simulink model ""  (R2025b)
settings: Solver=FixedStepAuto  StartTime=0.0  StopTime=inf  FixedStep=0.01  RelTol=1e-3
undefined symbols (not defined in the file or in its folder): LF
libraries: instrumentseriallib x4, simulink x1
settings Model: Creator=talles  LastModifiedBy=a_jax

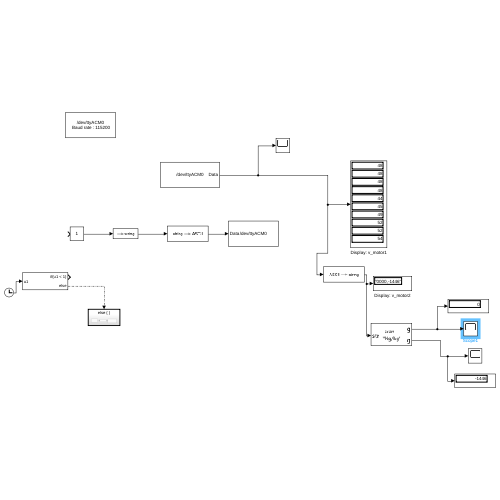
[thumbnail: Simulink's stored preview of the top-level diagram]
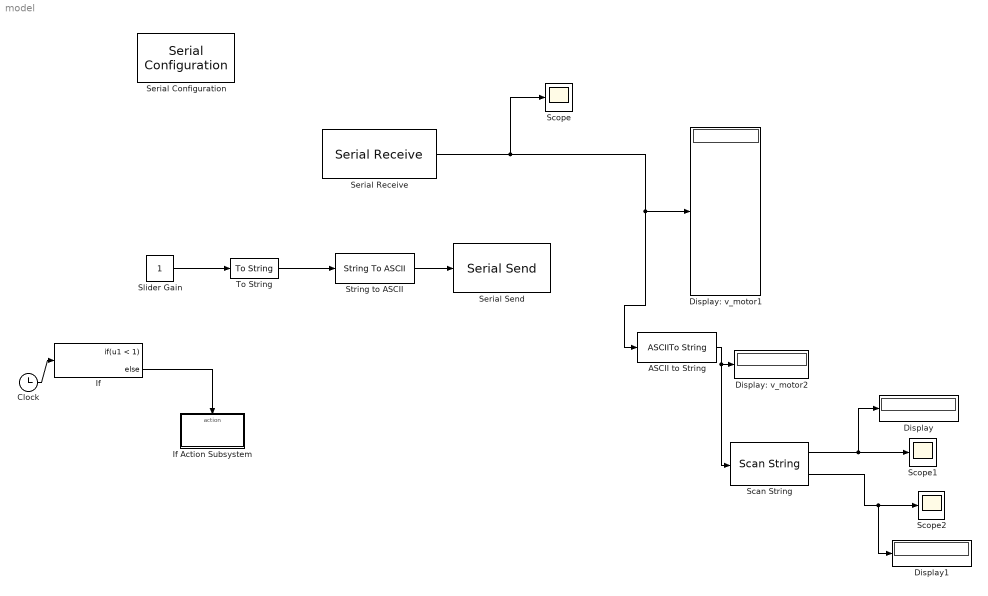
== system model ==
  ASCII to String : ASCIIToString
  Clock : Clock
  Display : Display
  Display1 : Display
  Display: v_motor1 : Display
      settings: Decimation=50
  Display: v_motor2 : Display
      settings: Decimation=50
  If : If  IfExpression=u1 < 1
  If Action Subsystem : Subsystem  TreatAsAtomicUnit=on
  Scan String : ScanString  Format="\"%g,%g\""
  Scope : Scope
      settings: ActiveDisplayYMinimum=4.625  ActiveDisplayYMaximum=58.375
  Scope1 : Scope
      settings: ActiveDisplayYMinimum=-384.80010076421058  ActiveDisplayYMaximum=1281.9889306839898
  Scope2 : Scope
      settings: ActiveDisplayYMinimum=-1626.75  ActiveDisplayYMaximum=180.74999999999997  DataLoggingVariableName=ScopeData2
  Serial Configuration : instrumentseriallib/Serial Configuration  Priority=-200000  PortSel=/dev/ttyACM0  Port=/dev/ttyACM0  ComPort=/dev/ttyACM0  BaudRate=115200  DataBits=8  Parity=none  StopBits=1  ByteOrder=little-endian  FlowControl=none  Timeout=0.0001  SimulateUsing=Interpreted execution  BlockInModel=on  aMode=1
      settings: LibrarySourceBlock=embeddedtargetslib/Host Communication/Serial Configuration
  Serial Receive : instrumentseriallib/Serial Receive  Priority=1  PortSel=/dev/ttyACM0  Port=/dev/ttyACM0  ComPort=/dev/ttyACM0  DataType=uint8  SaveDataType=uint8  ToggleHeader=on  Header=[10]  ToggleDataSize=on  DataSize=[10 1]  ToggleTerminator=off  Terminator=LF ('\n')  CustomTerminator=[]  InputFormat=Column major  EnableBlockingMode=on  ActionDataUnavailable=Output last received value  ActionWhenDataUnavailable=Output last received value  CustomValue=0  SampleTime=0.01  SimulateUsing=Interpreted execution  BlockInModel=on  aMode=1  LibraryInUse=instrumentlib
  Serial Send : instrumentseriallib/Serial Send  Priority=1  PortSel=/dev/ttyACM0  Port=/dev/ttyACM0  ComPort=/dev/ttyACM0  Header=[10]  Terminator=<none>  CustomTerminator=[]  EnableBlockingMode=on  SimulateUsing=Interpreted execution  BlockInModel=on  aMode=1
      settings: LibrarySourceBlock=embeddedtargetslib/Host Communication/Serial Send
  Slider Gain : simulink/Math Operations/Slider Gain  gain=1  low=-5  high=5
  String to ASCII : StringToASCII
  To String : ToString
  wires:
  ASCII to String/1 -> Scan String/1, Display: v_motor2/1
  Serial Receive/1 -> Scope/1, ASCII to String/1, Display: v_motor1/1
  Clock/1 -> If/1
  If/2 -> If Action Subsystem/Action
  To String/1 -> String to ASCII/1
  Scan String/1 -> Display/1, Scope1/1
  Scan String/2 -> Display1/1, Scope2/1
  Slider Gain/1 -> To String/1
  String to ASCII/1 -> Serial Send/1

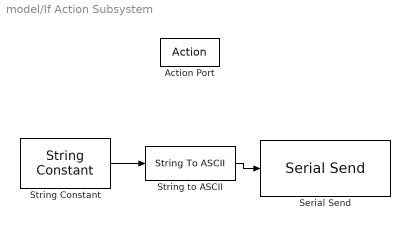
== system model/If Action Subsystem ==
  Action Port : ActionPort  ActionPortLabel=else
  Serial Send : instrumentseriallib/Serial Send  Priority=1  PortSel=/dev/ttyACM0  Port=/dev/ttyACM0  ComPort=/dev/ttyACM0  Header=[]  Terminator=LF ('\n')  CustomTerminator=[]  EnableBlockingMode=on  SimulateUsing=Interpreted execution  BlockInModel=on  aMode=1
  String Constant : StringConstant  String="\"1111,5556\""
  String to ASCII : StringToASCII
  wires:
  String Constant/1 -> String to ASCII/1
  String to ASCII/1 -> Serial Send/1
